simulink model "iio_sys_obj_sim"  (R2013b)
settings: Solver=ode45  StartTime=0.0  StopTime=10  RelTol=1e-3
undefined symbols (not defined in the file or in its folder): ad9361, cf, lpc
settings Model: Creator=ACozma  LastModifiedBy=ACozma

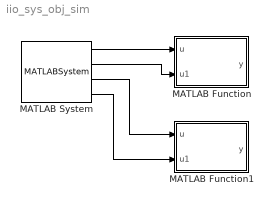
== system iio_sys_obj_sim ==
  MATLAB Function : MATLAB Function  TreatAsAtomicUnit=on  SystemSampleTime=1
  MATLAB Function1 : MATLAB Function  TreatAsAtomicUnit=on  SystemSampleTime=1
  MATLAB System : MATLABSystem  System=iio_sys_obj  SimulateUsing=Interpreted execution  ip_address=192.168.1.142  dev_name=cf-ad9361-lpc  ch_size=8192  ch_no=4
      mask Type: iio_sys_obj
      mask Display: disp('iio_sys_obj');
  wires:
  MATLAB System/1 -> MATLAB Function/1(u)
  MATLAB System/2 -> MATLAB Function/2(u1)
  MATLAB System/3 -> MATLAB Function1/1(u)
  MATLAB System/4 -> MATLAB Function1/2(u1)

== matlab function iio_sys_obj_sim/MATLAB Function1 ==
  data: u input; y output; u1 input
function y = fcn(u, u1)
%#codegen

%generate a complex output signal
y = complex(u, u1);

%compute the FFT
sample_rate = 30720000;
num_samples = length(y);
f = -sample_rate/2:sample_rate/(num_samples):sample_rate/2;
signal1 = y;
Nsignal = length(y);
%w = hamming(Nsignal);
%newsignal1 = signal1.*w;
newsignal1 = signal1;
fdata1 = 20*log10(abs(fftshift(fft(newsignal1), Nsignal)))/Nsignal;

figure(2); 
subplot(211); plot(1:1:length(u), u, 1:1:length(u1), u1); grid

subplot(212); plot(f(1:end-1), fdata1); grid(); xlim([f(1) f(end)]); ylim([min(fdata1)*1.1 max(fdata1)*1.1]);

== matlab function iio_sys_obj_sim/MATLAB Function ==
  data: u input; y output; u1 input
function y = fcn(u, u1)
%#codegen

%generate a complex output signal
y = complex(u, u1);

%compute the FFT
sample_rate = 30720000;
num_samples = length(y);
f = -sample_rate/2:sample_rate/(num_samples):sample_rate/2;
signal1 = y;
Nsignal = length(y);
%w = hamming(Nsignal);
%newsignal1 = signal1.*w;
newsignal1 = signal1;
fdata1 = 20*log10(abs(fftshift(fft(newsignal1), Nsignal)))/Nsignal;

figure(1); 
subplot(211); plot(1:1:length(u), u, 1:1:length(u1), u1); grid

subplot(212); plot(f(1:end-1), fdata1); grid(); xlim([f(1) f(end)]); ylim([min(fdata1)*1.1 max(fdata1)*1.1]);
